simulink model "UAV_attitude_dynamics"  (R2016a)
settings: Solver=VariableStepAuto  StartTime=0.0  StopTime=10.0  RelTol=1e-3
values from neighbouring files (symbols this model uses):
  q0 = [1;0;0;0]    [init_UAV_model.m]
settings Model: Creator=mgreiff  LastModifiedBy=mgreiff

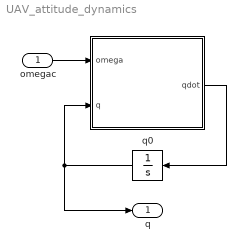
== system UAV_attitude_dynamics ==
  omegac : Inport  PortDimensions=3
  " " : MATLAB Function  TreatAsAtomicUnit=on
  q0 : Integrator  InitialCondition=q0
  q : Outport  PortDimensions=4
  wires:
  " "/1(qdot) -> q0/1
  q0/1 -> " "/2(q), q/1
  omegac/1 -> " "/1(omega)

== matlab function UAV_attitude_dynamics/  ==
  data: omega input; q input; qdot output
function qdot  = f(omega, q)
% ~~~ Copyright (c) 2018 Marcus Greiff (see LICENCE.md) ~~~
%
% Model of the attitude rate dynamics, a subset of the UAV dynamics
%
%    qdot  = f(omega, q)
%
% Omega is the attitude rate defined with respect to the global frame of
% reference and q denotes a quaternion in a Cayleigh-Dickinson construction
% with the Hamilton convention (right-handed).

% Normalize quaternion
q = q/norm(q);
qw = q(1);
qv = q(2:4);

% Quaternion derivative
qdot = zeros(4,1);
qdot(1)   = 0.5 * -qv'*omega;
qdot(2:4) = 0.5 * (qw*omega + cross(qv, omega));
end
